simulink model "tst3"  (R2013b)
settings: Solver=VariableStepDiscrete  StartTime=0.0  StopTime=StopTime  RelTol=1e-3
values from neighbouring files (symbols this model uses):
  fs = 256e3    (= 256000)    [design_2ord_sc_sigma_delta_adc_20211008.m]    (also in run_limited_bit_width_sum.m; run_limited_bit_width_sum_enob.m; run_tst1.m)
  osr1 = 2^16    (= 65536)    [run_tst1.m]
settings Model: Creator=eric  LastModifiedBy=eric

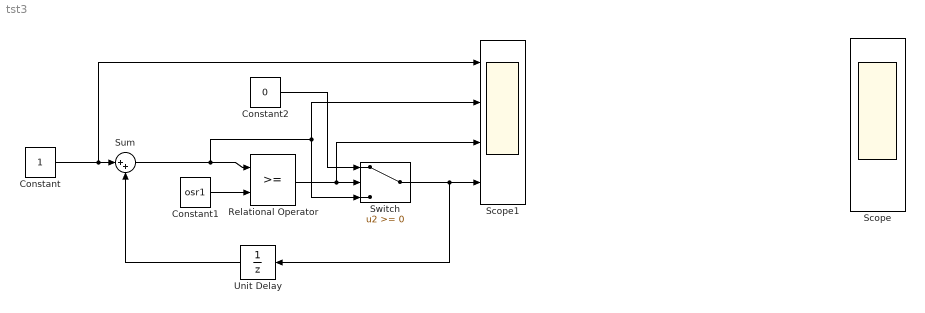
== system tst3 ==
  Constant : Constant  SampleTime=1/fs
  Constant1 : Constant  Value=osr1  SampleTime=1/fs
  Constant2 : Constant  Value=0  SampleTime=1/fs
  Relational Operator : RelationalOperator  OutDataTypeStr=boolean  SampleTime=1/fs
  Scope : Scope  NumInputPorts=4
      settings: TimeRange=0.02  YMin=0.89999997~0.8~-0.2~-1  YMax=0.90000003~2~0.8~1  MaxDataPoints=20000
  Scope1 : Scope  NumInputPorts=4
      settings: YMin=-5~-0.5~-5~-5  YMax=5~1.5~5~5
  Sum : Sum  Inputs=|++  SampleTime=1/fs
  Switch : Switch  SampleTime=1/fs
  Unit Delay : UnitDelay  SampleTime=1/fs
  wires:
  Constant1/1 -> Relational Operator/2
  Sum/1 -> Switch/3, Scope1/2, Relational Operator/1
  Constant2/1 -> Switch/1
  Relational Operator/1 -> Scope1/3, Switch/2
  Constant/1 -> Scope1/1, Sum/1
  Switch/1 -> Scope1/4, Unit Delay/1
  Unit Delay/1 -> Sum/2
